simulink model "smith"  (R2019a)
settings: Solver=ode4  StartTime=0.0  StopTime=endtime  FixedStep=0.001  RelTol=1e-3
values from neighbouring files (symbols this model uses):
  bike_m = bike    [Untitled2.m]
undefined symbols (not defined in the file or in its folder): K2
settings Model: Creator=chris  LastModifiedBy=chris

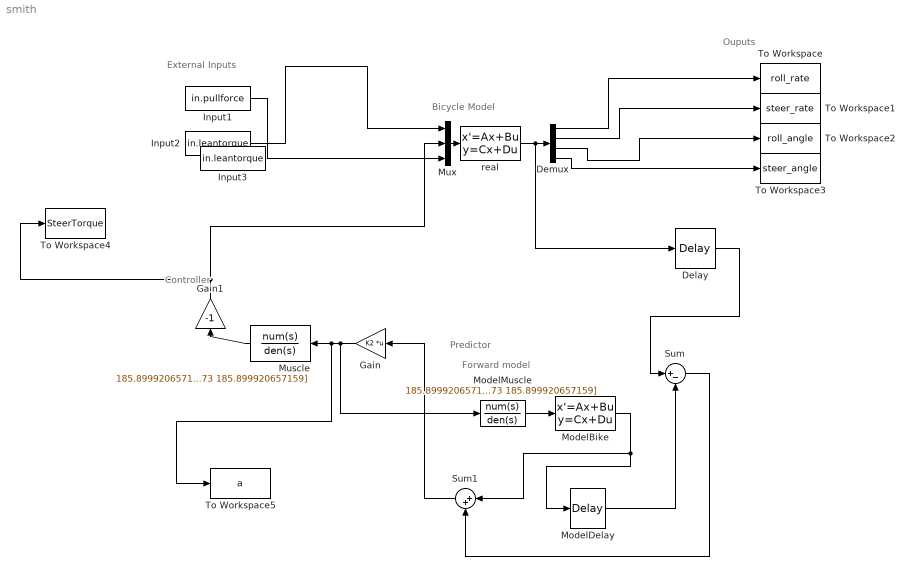
== system smith ==
  note: Bicycle Model
  note: External Inputs
  note: Controller
  note: Ouputs
  note: Predictor
  note: Forward model
  " ModelDelay " : TransportDelay  DelayTime=0.025
  Delay : TransportDelay  DelayTime=0.025
  Demux : Demux
  Gain : Gain  Gain=K2  Multiplication=Matrix(K*u) (u vector)
  Gain1 : Gain  Gain=-1
  Input1 : FromWorkspace  VariableName=in.pullforce  SampleTime=0
  Input2 : FromWorkspace  VariableName=in.leantorque  SampleTime=0
  Input3 : FromWorkspace  VariableName=in.leantorque  SampleTime=0
  "ModelBike " : StateSpace  A=bike_m.A  B=bike_m.B(:,2)  C=[1 0 0 0;0 1 0 0;0 0 1 0;0 0 0 1]  D=[0;0;0;0]  InitialCondition=0
  ModelMuscle : TransferFcn  Numerator=185.899920657159  Denominator=[1 19.2821119516073 185.899920657159]
  Muscle : TransferFcn  Numerator=185.899920657159  Denominator=[1 19.2821119516073 185.899920657159]
  Mux : Mux  Inputs=3
  Sum : Sum  Inputs=|+-
  Sum1 : Sum  Inputs=|++
  To Workspace : ToWorkspace  VariableName=roll_rate  SampleTime=-1
  To Workspace1 : ToWorkspace  VariableName=steer_rate  SampleTime=-1
  To Workspace2 : ToWorkspace  VariableName=roll_angle  SampleTime=-1
  To Workspace3 : ToWorkspace  VariableName=steer_angle  SampleTime=-1
  To Workspace4 : ToWorkspace  VariableName=SteerTorque  SampleTime=-1
  To Workspace5 : ToWorkspace  VariableName=a  SampleTime=-1
  "real " : StateSpace  A=bike_m.A  B=bike_m.B  C=bike_m.C  D=bike_m.D  InitialCondition=0
  wires:
  Gain/1 -> ModelMuscle/1, To Workspace5/1, Muscle/1
  Gain1/1 -> Mux/2, To Workspace4/1
  Input1/1 -> Mux/3
  Mux/1 -> "real "/1
  Demux/1 -> To Workspace/1
  Demux/2 -> To Workspace1/1
  Demux/3 -> To Workspace2/1
  Demux/4 -> To Workspace3/1
  Input2/1 -> Mux/1
  Muscle/1 -> Gain1/1
  ModelMuscle/1 -> "ModelBike "/1
  Delay/1 -> Sum/1
  "ModelBike "/1 -> " ModelDelay "/1, Sum1/1
  " ModelDelay "/1 -> Sum/2
  Sum/1 -> Sum1/2
  Sum1/1 -> Gain/1
  "real "/1 -> Delay/1, Demux/1
